simulink library "libturbines"  (R2025b)
settings: Solver=ode45  StartTime=0.0  StopTime=10.0  RelTol=1e-3  EnableMultiTasking=on
undefined symbols (not defined in the file): DiscIntNeverNeededParam, dt, faultOptions, noiseFlag
libraries: simulink x57, $bdroot x3
(part 1 of 5)
settings Model: Creator=grunnet  LastModifiedBy=yerai
settings SolverCC: AlgebraicLoopSolver=TrustRegion
settings DataIOCC: LimitDataPoints=on  SaveFormat=Array  SignalLoggingSaveFormat=ModelDataLogs  ReturnWorkspaceOutputs=off
settings OptimizationCC: ExpressionDepthLimit=2147483647.0  LifeSpan=inf
settings DebuggingCC: UnderspecifiedInitializationDetection=Classic  MergeDetectMultiDrivingBlocksExec=none  SolverPrmCheckMsg=warning  FcnCallInpInsideContextMsg=warning  UnconnectedInputMsg=warning  UnconnectedOutputMsg=warning  UnconnectedLineMsg=warning  StateNameClashWarn=warning  SFUnexpectedBacktrackingDiag=warning  SFNoUnconditionalDefaultTransitionDiag=warning  SFExecutionAtInitializationDiag=none  ArithmeticOperatorsInVariantConditions=warning
settings HardwareCC: ProdBitPerPointer=32.0  ProdBitPerSizeT=32.0  ProdBitPerPtrDiffT=32.0  ProdLargestAtomicFloat=None  ProdIntDivRoundTo=Undefined  ProdEndianess=Unspecified  ProdWordSize=32.0  ProdHWDeviceType=32-bit Generic
settings ModelReferenceCC: EnableRefExpFcnMdlSchedulingChecks=on  PropagateSignalLabelsOutOfModel=off
settings SFSimCC: SimUseLocalCustomCode=off  CustomCodeUndefinedFunction=UseInterfaceOnly
settings RTWCC: RTWUseLocalCustomCode=off  GPUComputeCapability=3.5  DLArmComputeVersion=19.05
settings CodeAppCC: StateflowObjectComments=on
settings GRTTargetCC: TargetLangStandard=C89/C90 (ANSI)  CombineOutputUpdateFcns=off  GRTInterface=on
settings ConfigComp: CovMetricSettings=dw  CovSaveCumulativeToWorkspaceVar=on  CovSaveSingleToWorkspaceVar=on  CovExternalEMLEnable=off

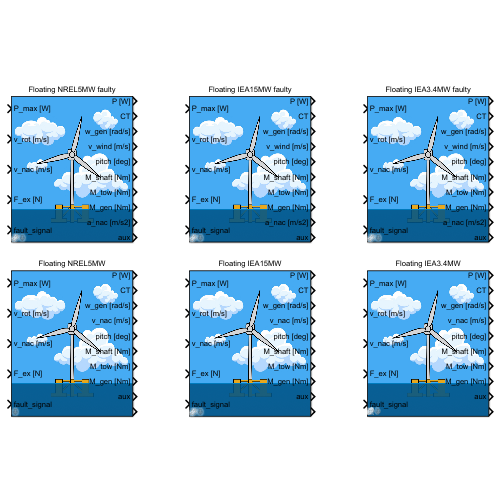
[thumbnail: Simulink's stored preview of the top-level diagram]
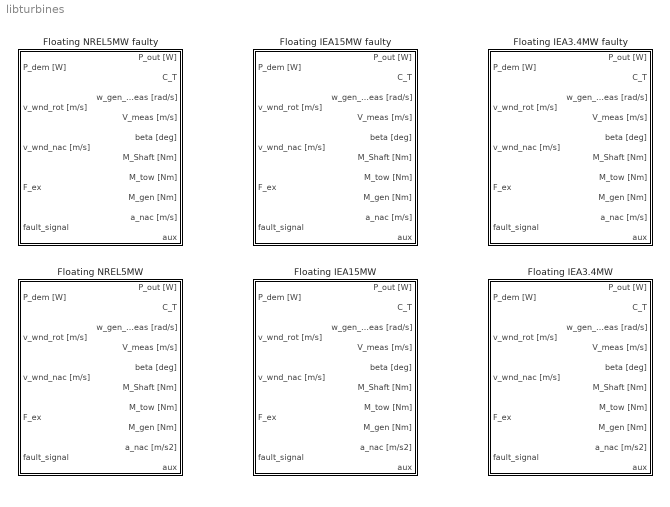
== system libturbines ==
  Floating IEA15MW : Subsystem  AncestorBlock=libturbines/Floating NREL5MW  mask(Wind Turbine){w_gen_ini=0.78788, beta_ini=0, auto=on, torq_ini=0}
      mask prompts: w_gen_ini "Initial generator velocity  [rad/s]"; beta_ini "Initial blade pitch [degrees]"; auto "Auto initial torque"; torq_ini "Initial generator torque"
      mask help: NREL 5MW Virtual Turbine
      mask init:
      | % l = load(file);
      | l               = get_param(gcb,'UserData');
      | env             = l.env;
      | wt              = l.wt;
      | plat            = l.plat;
      | wt.ctrl.gen.ini = w_gen_ini;
      | 
      | 
      | if(auto)
      |     wt.ctrl.torq.ini = min(interp1(wt.ctrl.torq.wg,wt.ctrl.torq.M,w_gen_ini,'spline'),wt.ctrl.torq.lim);
      | else
      |     wt.ctrl.torq.ini = torq_ini;
      | end
      | 
      | wt.pitch.ini        = beta_ini;
      | wt.ctrl.pitch.ini   = beta_ini;
      | wt.gen.torq.ini     = wt.ctrl.torq.ini;
      | wt.gen.ini          = w_gen_ini;
      | wt.rotor.ini        = w_gen_ini/wt.gen.N;
      mask Display:
      | image('FOWT.png');
      | 
      | port_label('output',1,'P [W]')
      | port_label('output',2,'CT')
      | port_label('output',3,'w_gen [rad/s]')
      | port_label('output',4,'v_nac [m/s]')
      | port_label('output',5,'pitch [deg]')
      | port_label('output',6,'M_shaft [Nm]')
      | port_label('output',7,'M_tow [Nm]')
      | port_label('output',8,'M_gen [Nm]')
      | port_label('output',9,'aux')
      | 
      | port_label('input',1,'P_max [W]')
      | port_label('input',2,'v_rot [m/s]')
      | port_label('input',3,'v_nac [m/s]')
      | port_label('input',4,'F_ex [N]')
      | port_label('input',5,'fault_signal')
  Floating IEA15MW faulty : Subsystem  AncestorBlock=libturbines/Floating NREL5MW faulty  mask(Wind Turbine){w_gen_ini=0.78788, beta_ini=0, auto=on, torq_ini=0}
      mask prompts: w_gen_ini "Initial generator velocity  [rad/s]"; beta_ini "Initial blade pitch [degrees]"; auto "Auto initial torque"; torq_ini "Initial generator torque"
      mask help: NREL 5MW Virtual Turbine
      mask init: same as libturbines/Floating IEA15MW
      mask Display:
      | image('FOWT.png');
      | 
      | port_label('output',1,'P [W]')
      | port_label('output',2,'CT')
      | port_label('output',3,'w_gen [rad/s]')
      | port_label('output',4,'v_wind [m/s]')
      | port_label('output',5,'pitch [deg]')
      | port_label('output',6,'M_shaft [Nm]')
      | port_label('output',7,'M_tow [Nm]')
      | port_label('output',8,'M_gen [Nm]')
      | port_label('output',9,'a_nac [m/s2]')
      | port_label('output',10,'aux')
      | 
      | port_label('input',1,'P_max [W]')
      | port_label('input',2,'v_rot [m/s]')
      | port_label('input',3,'v_nac [m/s]')
      | port_label('input',4,'F_ex [N]')
      | port_label('input',5,'fault_signal')
  Floating IEA3.4MW : Subsystem  AncestorBlock=libturbines/Floating IEA15MW  mask(Wind Turbine){w_gen_ini=118.1754, beta_ini=0, auto=on, torq_ini=0}
      mask prompts: w_gen_ini "Initial generator velocity  [rad/s]"; beta_ini "Initial blade pitch [degrees]"; auto "Auto initial torque"; torq_ini "Initial generator torque"
      mask help: NREL 5MW Virtual Turbine
      mask init: same as libturbines/Floating IEA15MW
      mask Display:
      | image('FOWT.png');
      | 
      | port_label('output',1,'P [W]')
      | port_label('output',2,'CT')
      | port_label('output',3,'w_gen [rad/s]')
      | port_label('output',4,'v_nac [m/s]')
      | port_label('output',5,'pitch [deg]')
      | port_label('output',6,'M_shaft [Nm]')
      | port_label('output',7,'M_tow [Nm]')
      | port_label('output',8,'M_gen [Nm]')
      | port_label('output',9,'aux')
      | 
      | port_label('input',1,'P_max [W]')
      | port_label('input',2,'v_rot [m/s]')
      | port_label('input',3,'v_nac [m/s]')
      | port_label('input',4,'F_ex [N]')
      | port_label('input',5,'fault_signal')
  Floating IEA3.4MW faulty : Subsystem  AncestorBlock=libturbines/Floating IEA15MW faulty  mask(Wind Turbine){w_gen_ini=118.1754, beta_ini=0, auto=on, torq_ini=0}
      mask prompts: w_gen_ini "Initial generator velocity  [rad/s]"; beta_ini "Initial blade pitch [degrees]"; auto "Auto initial torque"; torq_ini "Initial generator torque"
      mask help: NREL 5MW Virtual Turbine
      mask init: same as libturbines/Floating IEA15MW
      mask Display:
      | image('FOWT.png');
      | 
      | port_label('output',1,'P [W]')
      | port_label('output',2,'CT')
      | port_label('output',3,'w_gen [rad/s]')
      | port_label('output',4,'v_wind [m/s]')
      | port_label('output',5,'pitch [deg]')
      | port_label('output',6,'M_shaft [Nm]')
      | port_label('output',7,'M_tow [Nm]')
      | port_label('output',8,'M_gen [Nm]')
      | port_label('output',9,'a_nac [m/s2]')
      | port_label('output',10,'aux')
      | 
      | port_label('input',1,'P_max [W]')
      | port_label('input',2,'v_rot [m/s]')
      | port_label('input',3,'v_nac [m/s]')
      | port_label('input',4,'F_ex [N]')
      | port_label('input',5,'fault_signal')
  Floating NREL5MW : Subsystem  mask(Wind Turbine){w_gen_ini=50, beta_ini=0, auto=off, torq_ini=0}
      mask prompts: w_gen_ini "Initial generator velocity  [rad/s]"; beta_ini "Initial blade pitch [degrees]"; auto "Auto initial torque"; torq_ini "Initial generator torque"
      mask help: NREL 5MW Virtual Turbine
      mask init: same as libturbines/Floating IEA15MW
      mask Display:
      | image('FOWT.png');
      | 
      | port_label('output',1,'P [W]')
      | port_label('output',2,'CT')
      | port_label('output',3,'w_gen [rad/s]')
      | port_label('output',4,'v_nac [m/s]')
      | port_label('output',5,'pitch [deg]')
      | port_label('output',6,'M_shaft [Nm]')
      | port_label('output',7,'M_tow [Nm]')
      | port_label('output',8,'M_gen [Nm]')
      | port_label('output',9,'aux')
      | 
      | port_label('input',1,'P_max [W]')
      | port_label('input',2,'v_rot [m/s]')
      | port_label('input',3,'v_nac [m/s]')
      | port_label('input',4,'F_ex [N]')
      | port_label('input',5,'fault_signal')
  Floating NREL5MW faulty : Subsystem  AncestorBlock=libturbines/Faulty NREL5MW  mask(Wind Turbine){w_gen_ini=50, beta_ini=0, auto=off, torq_ini=0}
      mask prompts: w_gen_ini "Initial generator velocity  [rad/s]"; beta_ini "Initial blade pitch [degrees]"; auto "Auto initial torque"; torq_ini "Initial generator torque"
      mask help: NREL 5MW Virtual Turbine
      mask init: same as libturbines/Floating IEA15MW
      mask Display:
      | image('FOWT.png');
      | 
      | port_label('output',1,'P [W]')
      | port_label('output',2,'CT')
      | port_label('output',3,'w_gen [rad/s]')
      | port_label('output',4,'v_wind [m/s]')
      | port_label('output',5,'pitch [deg]')
      | port_label('output',6,'M_shaft [Nm]')
      | port_label('output',7,'M_tow [Nm]')
      | port_label('output',8,'M_gen [Nm]')
      | port_label('output',9,'a_nac [m/s2]')
      | port_label('output',10,'aux')
      | 
      | port_label('input',1,'P_max [W]')
      | port_label('input',2,'v_rot [m/s]')
      | port_label('input',3,'v_nac [m/s]')
      | port_label('input',4,'F_ex [N]')
      | port_label('input',5,'fault_signal')

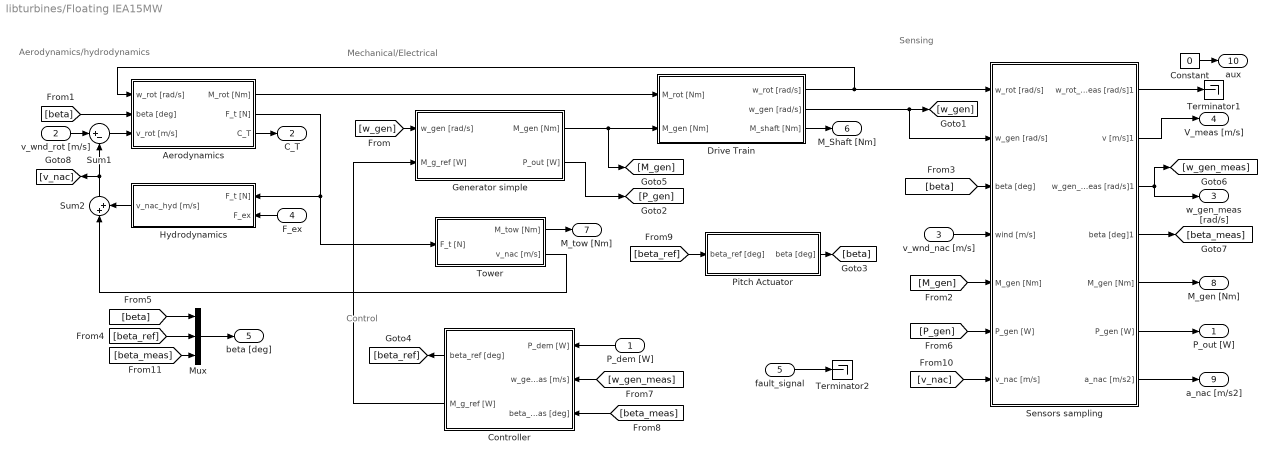
== system libturbines/Floating IEA15MW ==
  note: Control
  note: Aerodynamics/hydrodynamics
  note: Mechanical/Electrical
  note: Sensing
  P_dem [W] : Inport
  v_wnd_rot [m/s] : Inport  Port=2
  v_wnd_nac [m/s] : Inport  Port=3
  F_ex : Inport  Port=4
  fault_signal : Inport  Port=5
  Aerodynamics : Subsystem
  Constant : Constant  Value=0
  Controller : Subsystem
  Drive Train : Subsystem
  Generator simple : Subsystem
  Hydrodynamics : Subsystem
  Mux : Mux  Inputs=3
  Pitch Actuator : Subsystem
  Sensors sampling : Subsystem
  Sum1 : Sum  Inputs=|+-  InputSameDT=on  SaturateOnIntegerOverflow=on  OutDataTypeStr=Inherit: Same as first input
  Sum2 : Sum  Inputs=|++  InputSameDT=on  SaturateOnIntegerOverflow=on  OutDataTypeStr=Inherit: Same as first input
  Terminator1 : Terminator
  Terminator2 : Terminator
  "Tower " : Subsystem
  P_out [W] : Outport
  C_T : Outport  Port=2
  w_gen_meas [rad/s] : Outport  Port=3
  V_meas [m/s] : Outport  Port=4
  beta [deg] : Outport  Port=5
  M_Shaft [Nm] : Outport  Port=6
  M_tow [Nm] : Outport  Port=7
  M_gen [Nm] : Outport  Port=8
  a_nac [m/s2] : Outport  Port=9
  aux : Outport  Port=10
  wires:
  Sensors sampling/7(a_nac [m/s2]) -> a_nac [m/s2]/1
  [v_nac] -> Sensors sampling/7("v_nac [m/s] ")
  "Tower "/2(v_nac [m/s]) -> Sum2/1
  Sum2/1 -> Sum1/2, [v_nac]
  Hydrodynamics/1(v_nac_hyd [m/s]) -> Sum2/2
  [P_gen] -> Sensors sampling/6("P_gen [W] ")
  [M_gen] -> Sensors sampling/5("M_gen [Nm] ")
  Generator simple/2(P_out [W]) -> [P_gen]
  Sensors sampling/6(P_gen [W]) -> P_out [W]/1
  Sensors sampling/5(M_gen [Nm]) -> M_gen [Nm]/1
  Sensors sampling/4(beta [deg]1) -> [beta_meas]
  Sensors sampling/3(w_gen_meas [rad/s]1) -> [w_gen_meas], w_gen_meas [rad/s]/1
  Sensors sampling/2(v [m/s]1) -> V_meas [m/s]/1
  Sensors sampling/1(w_rot_meas [rad/s]1) -> Terminator1/1
  [beta] -> Aerodynamics/2(beta [deg])
  [w_gen] -> Generator simple/1(w_gen [rad/s])
  fault_signal/1 -> Terminator2/1
  Drive Train/3(M_shaft [Nm]) -> M_Shaft [Nm]/1
  v_wnd_nac [m/s]/1 -> Sensors sampling/4(wind [m/s])
  v_wnd_rot [m/s]/1 -> Sum1/1
  "Tower "/1(M_tow [Nm]) -> M_tow [Nm]/1
  Aerodynamics/2(F_t [N]) -> Hydrodynamics/1(F_t [N]), "Tower "/1(F_t [N])
  Pitch Actuator/1(beta [deg]) -> [beta]
  Controller/1(beta_ref [deg]) -> [beta_ref]
  P_dem [W]/1 -> Controller/1(P_dem [W])
  Controller/2(M_g_ref [W]) -> Generator simple/2(M_g_ref [W])
  Sum1/1 -> Aerodynamics/3(v_rot [m/s])
  Drive Train/2(w_gen [rad/s]) -> [w_gen], Sensors sampling/2(w_gen [rad/s])
  Generator simple/1(M_gen [Nm]) -> Drive Train/2(M_gen [Nm]), [M_gen]
  Drive Train/1(w_rot [rad/s]) -> Aerodynamics/1(w_rot [rad/s]), Sensors sampling/1("w_rot [rad/s] ")
  Aerodynamics/1(M_rot [Nm]) -> Drive Train/1(M_rot [Nm])
  Aerodynamics/3(C_T) -> C_T/1
  [beta] -> Sensors sampling/3("beta [deg] ")
  [beta_ref] -> Mux/2
  [beta] -> Mux/1
  [w_gen_meas] -> Controller/2(w_gen_meas [m/s])
  [beta_meas] -> Controller/3(beta_meas [deg])
  [beta_ref] -> Pitch Actuator/1(beta_ref [deg])
  [beta_meas] -> Mux/3
  F_ex/1 -> Hydrodynamics/2(F_ex)
  Mux/1 -> beta [deg]/1
  Constant/1 -> aux/1

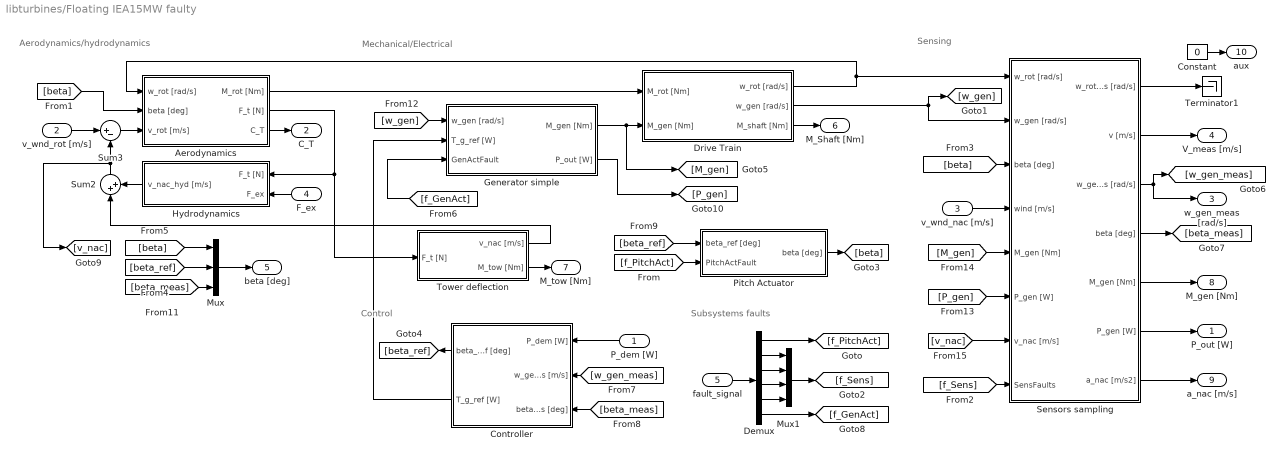
== system libturbines/Floating IEA15MW faulty ==
  note: Subsystems faults
  note: Sensing
  note: Mechanical/Electrical
  note: Aerodynamics/hydrodynamics
  note: Control
  P_dem [W] : Inport
  v_wnd_rot [m/s] : Inport  Port=2
  v_wnd_nac [m/s] : Inport  Port=3
  F_ex : Inport  Port=4
  fault_signal : Inport  Port=5
  Aerodynamics : Subsystem
  Constant : Constant  Value=0
  Controller : Subsystem
  Demux : Demux  Outputs=6
  Drive Train : Subsystem
  Generator simple : Subsystem
  Hydrodynamics : Subsystem
  Mux : Mux  Inputs=3
  Mux1 : Mux
  Pitch Actuator : Subsystem
  Sensors sampling : Subsystem
  Sum2 : Sum  Inputs=|++  InputSameDT=on  SaturateOnIntegerOverflow=on  OutDataTypeStr=Inherit: Same as first input
  Sum3 : Sum  Inputs=|+-  InputSameDT=on  SaturateOnIntegerOverflow=on  OutDataTypeStr=Inherit: Same as first input
  Terminator1 : Terminator
  "Tower deflection " : Subsystem
  P_out [W] : Outport
  C_T : Outport  Port=2
  w_gen_meas [rad/s] : Outport  Port=3
  V_meas [m/s] : Outport  Port=4
  beta [deg] : Outport  Port=5
  M_Shaft [Nm] : Outport  Port=6
  M_tow [Nm] : Outport  Port=7
  M_gen [Nm] : Outport  Port=8
  a_nac [m/s] : Outport  Port=9
  aux : Outport  Port=10
  wires:
  Demux/5 -> Mux1/4
  Demux/6 -> [f_GenAct]
  Sensors sampling/7(a_nac [m/s2]) -> a_nac [m/s]/1
  [v_nac] -> Sensors sampling/7("v_nac [m/s] ")
  "Tower deflection "/1(v_nac [m/s]) -> Sum2/1
  Sum2/1 -> Sum3/2, [v_nac]
  Hydrodynamics/1(v_nac_hyd [m/s]) -> Sum2/2
  v_wnd_rot [m/s]/1 -> Sum3/1
  Sum3/1 -> Aerodynamics/3(v_rot [m/s])
  [M_gen] -> Sensors sampling/5("M_gen [Nm] ")
  [P_gen] -> Sensors sampling/6("P_gen [W] ")
  Generator simple/2(P_out [W]) -> [P_gen]
  Sensors sampling/5(M_gen [Nm]) -> M_gen [Nm]/1
  Sensors sampling/6(P_gen [W]) -> P_out [W]/1
  [w_gen] -> Generator simple/1(w_gen [rad/s])
  [beta] -> Aerodynamics/2(beta [deg])
  Mux1/1 -> [f_Sens]
  Demux/4 -> Mux1/3
  Demux/2 -> Mux1/1
  Demux/3 -> Mux1/2
  Constant/1 -> aux/1
  Mux/1 -> beta [deg]/1
  F_ex/1 -> Hydrodynamics/2(F_ex)
  [beta_meas] -> Mux/3
  [beta_ref] -> Pitch Actuator/1(beta_ref [deg])
  [beta_meas] -> Controller/3(beta_meas [deg])
  [w_gen_meas] -> Controller/2(w_gen_meas [m/s])
  [f_GenAct] -> Generator simple/3(GenActFault)
  [beta] -> Mux/1
  [beta_ref] -> Mux/2
  [beta] -> Sensors sampling/3("beta [deg] ")
  [f_Sens] -> Sensors sampling/8(SensFaults)
  [f_PitchAct] -> Pitch Actuator/2(PitchActFault)
  Demux/1 -> [f_PitchAct]
  fault_signal/1 -> Demux/1
  Aerodynamics/3(C_T) -> C_T/1
  Aerodynamics/1(M_rot [Nm]) -> Drive Train/1(M_rot [Nm])
  Drive Train/1(w_rot [rad/s]) -> Sensors sampling/1("w_rot [rad/s] "), Aerodynamics/1(w_rot [rad/s])
  Generator simple/1(M_gen [Nm]) -> Drive Train/2(M_gen [Nm]), [M_gen]
  Drive Train/2(w_gen [rad/s]) -> Sensors sampling/2(w_gen [rad/s]), [w_gen]
  Sensors sampling/4(beta [deg]) -> [beta_meas]
  Sensors sampling/2(v [m/s]) -> V_meas [m/s]/1
  Controller/2(T_g_ref [W]) -> Generator simple/2(T_g_ref [W])
  Sensors sampling/3(w_gen_meas [rad/s]) -> [w_gen_meas], w_gen_meas [rad/s]/1
  P_dem [W]/1 -> Controller/1(P_dem [W])
  Controller/1(beta_ref [deg]) -> [beta_ref]
  Pitch Actuator/1(beta [deg]) -> [beta]
  Aerodynamics/2(F_t [N]) -> Hydrodynamics/1(F_t [N]), "Tower deflection "/1(F_t [N])
  "Tower deflection "/2(M_tow [Nm]) -> M_tow [Nm]/1
  v_wnd_nac [m/s]/1 -> Sensors sampling/4(wind [m/s])
  Drive Train/3(M_shaft [Nm]) -> M_Shaft [Nm]/1
  Sensors sampling/1(w_rot_meas [rad/s]) -> Terminator1/1

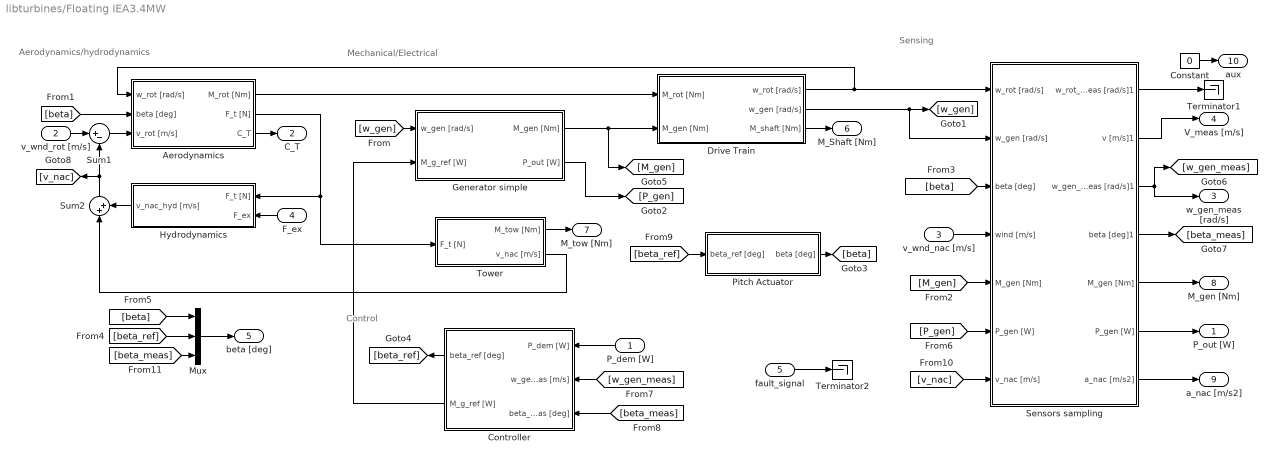
== system libturbines/Floating IEA3.4MW ==
  note: Control
  note: Aerodynamics/hydrodynamics
  note: Mechanical/Electrical
  note: Sensing
  P_dem [W] : Inport
  v_wnd_rot [m/s] : Inport  Port=2
  v_wnd_nac [m/s] : Inport  Port=3
  F_ex : Inport  Port=4
  fault_signal : Inport  Port=5
  Aerodynamics : Subsystem
  Constant : Constant  Value=0
  Controller : Subsystem
  Drive Train : Subsystem
  Generator simple : Subsystem
  Hydrodynamics : Subsystem
  Mux : Mux  Inputs=3
  Pitch Actuator : Subsystem
  Sensors sampling : Subsystem
  Sum1 : Sum  Inputs=|+-  InputSameDT=on  SaturateOnIntegerOverflow=on  OutDataTypeStr=Inherit: Same as first input
  Sum2 : Sum  Inputs=|++  InputSameDT=on  SaturateOnIntegerOverflow=on  OutDataTypeStr=Inherit: Same as first input
  Terminator1 : Terminator
  Terminator2 : Terminator
  "Tower " : Subsystem
  P_out [W] : Outport
  C_T : Outport  Port=2
  w_gen_meas [rad/s] : Outport  Port=3
  V_meas [m/s] : Outport  Port=4
  beta [deg] : Outport  Port=5
  M_Shaft [Nm] : Outport  Port=6
  M_tow [Nm] : Outport  Port=7
  M_gen [Nm] : Outport  Port=8
  a_nac [m/s2] : Outport  Port=9
  aux : Outport  Port=10
  wires:
  Sensors sampling/7(a_nac [m/s2]) -> a_nac [m/s2]/1
  [v_nac] -> Sensors sampling/7("v_nac [m/s] ")
  "Tower "/2(v_nac [m/s]) -> Sum2/1
  Sum2/1 -> Sum1/2, [v_nac]
  Hydrodynamics/1(v_nac_hyd [m/s]) -> Sum2/2
  [P_gen] -> Sensors sampling/6("P_gen [W] ")
  [M_gen] -> Sensors sampling/5("M_gen [Nm] ")
  Generator simple/2(P_out [W]) -> [P_gen]
  Sensors sampling/6(P_gen [W]) -> P_out [W]/1
  Sensors sampling/5(M_gen [Nm]) -> M_gen [Nm]/1
  Sensors sampling/4(beta [deg]1) -> [beta_meas]
  Sensors sampling/3(w_gen_meas [rad/s]1) -> [w_gen_meas], w_gen_meas [rad/s]/1
  Sensors sampling/2(v [m/s]1) -> V_meas [m/s]/1
  Sensors sampling/1(w_rot_meas [rad/s]1) -> Terminator1/1
  [beta] -> Aerodynamics/2(beta [deg])
  [w_gen] -> Generator simple/1(w_gen [rad/s])
  fault_signal/1 -> Terminator2/1
  Drive Train/3(M_shaft [Nm]) -> M_Shaft [Nm]/1
  v_wnd_nac [m/s]/1 -> Sensors sampling/4(wind [m/s])
  v_wnd_rot [m/s]/1 -> Sum1/1
  "Tower "/1(M_tow [Nm]) -> M_tow [Nm]/1
  Aerodynamics/2(F_t [N]) -> Hydrodynamics/1(F_t [N]), "Tower "/1(F_t [N])
  Pitch Actuator/1(beta [deg]) -> [beta]
  Controller/1(beta_ref [deg]) -> [beta_ref]
  P_dem [W]/1 -> Controller/1(P_dem [W])
  Controller/2(M_g_ref [W]) -> Generator simple/2(M_g_ref [W])
  Sum1/1 -> Aerodynamics/3(v_rot [m/s])
  Drive Train/2(w_gen [rad/s]) -> [w_gen], Sensors sampling/2(w_gen [rad/s])
  Generator simple/1(M_gen [Nm]) -> Drive Train/2(M_gen [Nm]), [M_gen]
  Drive Train/1(w_rot [rad/s]) -> Aerodynamics/1(w_rot [rad/s]), Sensors sampling/1("w_rot [rad/s] ")
  Aerodynamics/1(M_rot [Nm]) -> Drive Train/1(M_rot [Nm])
  Aerodynamics/3(C_T) -> C_T/1
  [beta] -> Sensors sampling/3("beta [deg] ")
  [beta_ref] -> Mux/2
  [beta] -> Mux/1
  [w_gen_meas] -> Controller/2(w_gen_meas [m/s])
  [beta_meas] -> Controller/3(beta_meas [deg])
  [beta_ref] -> Pitch Actuator/1(beta_ref [deg])
  [beta_meas] -> Mux/3
  F_ex/1 -> Hydrodynamics/2(F_ex)
  Mux/1 -> beta [deg]/1
  Constant/1 -> aux/1

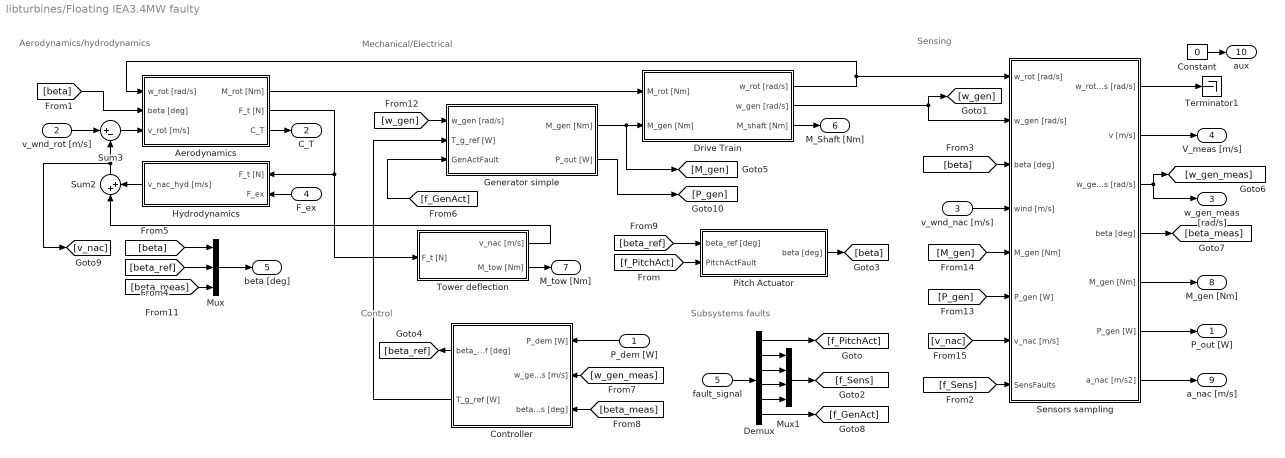
== system libturbines/Floating IEA3.4MW faulty ==
  note: Subsystems faults
  note: Sensing
  note: Mechanical/Electrical
  note: Aerodynamics/hydrodynamics
  note: Control
  P_dem [W] : Inport
  v_wnd_rot [m/s] : Inport  Port=2
  v_wnd_nac [m/s] : Inport  Port=3
  F_ex : Inport  Port=4
  fault_signal : Inport  Port=5
  Aerodynamics : Subsystem
  Constant : Constant  Value=0
  Controller : Subsystem
  Demux : Demux  Outputs=6
  Drive Train : Subsystem
  Generator simple : Subsystem
  Hydrodynamics : Subsystem
  Mux : Mux  Inputs=3
  Mux1 : Mux
  Pitch Actuator : Subsystem
  Sensors sampling : Subsystem
  Sum2 : Sum  Inputs=|++  InputSameDT=on  SaturateOnIntegerOverflow=on  OutDataTypeStr=Inherit: Same as first input
  Sum3 : Sum  Inputs=|+-  InputSameDT=on  SaturateOnIntegerOverflow=on  OutDataTypeStr=Inherit: Same as first input
  Terminator1 : Terminator
  "Tower deflection " : Subsystem
  P_out [W] : Outport
  C_T : Outport  Port=2
  w_gen_meas [rad/s] : Outport  Port=3
  V_meas [m/s] : Outport  Port=4
  beta [deg] : Outport  Port=5
  M_Shaft [Nm] : Outport  Port=6
  M_tow [Nm] : Outport  Port=7
  M_gen [Nm] : Outport  Port=8
  a_nac [m/s] : Outport  Port=9
  aux : Outport  Port=10
  wires:
  Demux/5 -> Mux1/4
  Demux/6 -> [f_GenAct]
  Sensors sampling/7(a_nac [m/s2]) -> a_nac [m/s]/1
  [v_nac] -> Sensors sampling/7("v_nac [m/s] ")
  "Tower deflection "/1(v_nac [m/s]) -> Sum2/1
  Sum2/1 -> Sum3/2, [v_nac]
  Hydrodynamics/1(v_nac_hyd [m/s]) -> Sum2/2
  v_wnd_rot [m/s]/1 -> Sum3/1
  Sum3/1 -> Aerodynamics/3(v_rot [m/s])
  [M_gen] -> Sensors sampling/5("M_gen [Nm] ")
  [P_gen] -> Sensors sampling/6("P_gen [W] ")
  Generator simple/2(P_out [W]) -> [P_gen]
  Sensors sampling/5(M_gen [Nm]) -> M_gen [Nm]/1
  Sensors sampling/6(P_gen [W]) -> P_out [W]/1
  [w_gen] -> Generator simple/1(w_gen [rad/s])
  [beta] -> Aerodynamics/2(beta [deg])
  Mux1/1 -> [f_Sens]
  Demux/4 -> Mux1/3
  Demux/2 -> Mux1/1
  Demux/3 -> Mux1/2
  Constant/1 -> aux/1
  Mux/1 -> beta [deg]/1
  F_ex/1 -> Hydrodynamics/2(F_ex)
  [beta_meas] -> Mux/3
  [beta_ref] -> Pitch Actuator/1(beta_ref [deg])
  [beta_meas] -> Controller/3(beta_meas [deg])
  [w_gen_meas] -> Controller/2(w_gen_meas [m/s])
  [f_GenAct] -> Generator simple/3(GenActFault)
  [beta] -> Mux/1
  [beta_ref] -> Mux/2
  [beta] -> Sensors sampling/3("beta [deg] ")
  [f_Sens] -> Sensors sampling/8(SensFaults)
  [f_PitchAct] -> Pitch Actuator/2(PitchActFault)
  Demux/1 -> [f_PitchAct]
  fault_signal/1 -> Demux/1
  Aerodynamics/3(C_T) -> C_T/1
  Aerodynamics/1(M_rot [Nm]) -> Drive Train/1(M_rot [Nm])
  Drive Train/1(w_rot [rad/s]) -> Sensors sampling/1("w_rot [rad/s] "), Aerodynamics/1(w_rot [rad/s])
  Generator simple/1(M_gen [Nm]) -> Drive Train/2(M_gen [Nm]), [M_gen]
  Drive Train/2(w_gen [rad/s]) -> Sensors sampling/2(w_gen [rad/s]), [w_gen]
  Sensors sampling/4(beta [deg]) -> [beta_meas]
  Sensors sampling/2(v [m/s]) -> V_meas [m/s]/1
  Controller/2(T_g_ref [W]) -> Generator simple/2(T_g_ref [W])
  Sensors sampling/3(w_gen_meas [rad/s]) -> [w_gen_meas], w_gen_meas [rad/s]/1
  P_dem [W]/1 -> Controller/1(P_dem [W])
  Controller/1(beta_ref [deg]) -> [beta_ref]
  Pitch Actuator/1(beta [deg]) -> [beta]
  Aerodynamics/2(F_t [N]) -> Hydrodynamics/1(F_t [N]), "Tower deflection "/1(F_t [N])
  "Tower deflection "/2(M_tow [Nm]) -> M_tow [Nm]/1
  v_wnd_nac [m/s]/1 -> Sensors sampling/4(wind [m/s])
  Drive Train/3(M_shaft [Nm]) -> M_Shaft [Nm]/1
  Sensors sampling/1(w_rot_meas [rad/s]) -> Terminator1/1

== system libturbines/Floating NREL5MW ==
  note: Sensing
  note: Mechanical/Electrical
  note: Aerodynamics/hydrodynamics
  note: Control
  P_dem [W] : Inport
  v_wnd_rot [m/s] : Inport  Port=2
  v_wnd_nac [m/s] : Inport  Port=3
  F_ex : Inport  Port=4
  fault_signal : Inport  Port=5
  Aerodynamics : Subsystem
  Constant : Constant  Value=0
  Controller : Subsystem
  Drive Train : Subsystem
  Generator simple : Subsystem
  Hydrodynamics : Subsystem
  Mux : Mux  Inputs=3
  Pitch Actuator : Subsystem
  Sensors sampling : Subsystem
  Sum1 : Sum  Inputs=|+-  InputSameDT=on  SaturateOnIntegerOverflow=on  OutDataTypeStr=Inherit: Same as first input
  Sum2 : Sum  Inputs=|++  InputSameDT=on  SaturateOnIntegerOverflow=on  OutDataTypeStr=Inherit: Same as first input
  Terminator1 : Terminator
  Terminator2 : Terminator
  "Tower " : Subsystem
  P_out [W] : Outport
  C_T : Outport  Port=2
  w_gen_meas [rad/s] : Outport  Port=3
  V_meas [m/s] : Outport  Port=4
  beta [deg] : Outport  Port=5
  M_Shaft [Nm] : Outport  Port=6
  M_tow [Nm] : Outport  Port=7
  M_gen [Nm] : Outport  Port=8
  a_nac [m/s2] : Outport  Port=9
  aux : Outport  Port=10
  wires:
  Constant/1 -> aux/1
  Mux/1 -> beta [deg]/1
  F_ex/1 -> Hydrodynamics/2(F_ex)
  [beta_meas] -> Mux/3
  [beta_ref] -> Pitch Actuator/1(beta_ref [deg])
  [beta_meas] -> Controller/3(beta_meas [deg])
  [w_gen_meas] -> Controller/2(w_gen_meas [m/s])
  [beta] -> Mux/1
  [beta_ref] -> Mux/2
  [beta] -> Sensors sampling/3("beta [deg] ")
  Aerodynamics/3(C_T) -> C_T/1
  Aerodynamics/1(M_rot [Nm]) -> Drive Train/1(M_rot [Nm])
  Drive Train/1(w_rot [rad/s]) -> Sensors sampling/1("w_rot [rad/s] "), Aerodynamics/1(w_rot [rad/s])
  Generator simple/1(M_gen [Nm]) -> [M_gen], Drive Train/2(M_gen [Nm])
  Drive Train/2(w_gen [rad/s]) -> Sensors sampling/2(w_gen [rad/s]), [w_gen]
  Sum1/1 -> Aerodynamics/3(v_rot [m/s])
  Controller/2(M_g_ref [W]) -> Generator simple/2(M_g_ref [W])
  P_dem [W]/1 -> Controller/1(P_dem [W])
  Controller/1(beta_ref [deg]) -> [beta_ref]
  Pitch Actuator/1(beta [deg]) -> [beta]
  Aerodynamics/2(F_t [N]) -> "Tower "/1(F_t [N]), Hydrodynamics/1(F_t [N])
  "Tower "/1(M_tow [Nm]) -> M_tow [Nm]/1
  v_wnd_rot [m/s]/1 -> Sum1/1
  v_wnd_nac [m/s]/1 -> Sensors sampling/4(wind [m/s])
  Drive Train/3(M_shaft [Nm]) -> M_Shaft [Nm]/1
  fault_signal/1 -> Terminator2/1
  [w_gen] -> Generator simple/1(w_gen [rad/s])
  [beta] -> Aerodynamics/2(beta [deg])
  Sensors sampling/1(w_rot_meas [rad/s]1) -> Terminator1/1
  Sensors sampling/2(v [m/s]1) -> V_meas [m/s]/1
  Sensors sampling/3(w_gen_meas [rad/s]1) -> w_gen_meas [rad/s]/1, [w_gen_meas]
  Sensors sampling/4(beta [deg]1) -> [beta_meas]
  Sensors sampling/5(M_gen [Nm]) -> M_gen [Nm]/1
  Sensors sampling/6(P_gen [W]) -> P_out [W]/1
  Generator simple/2(P_out [W]) -> [P_gen]
  [M_gen] -> Sensors sampling/5("M_gen [Nm] ")
  [P_gen] -> Sensors sampling/6("P_gen [W] ")
  Hydrodynamics/1(v_nac_hyd [m/s]) -> Sum2/2
  Sum2/1 -> [v_nac], Sum1/2
  "Tower "/2(v_nac [m/s]) -> Sum2/1
  [v_nac] -> Sensors sampling/7("v_nac [m/s] ")
  Sensors sampling/7(a_nac [m/s2]) -> a_nac [m/s2]/1

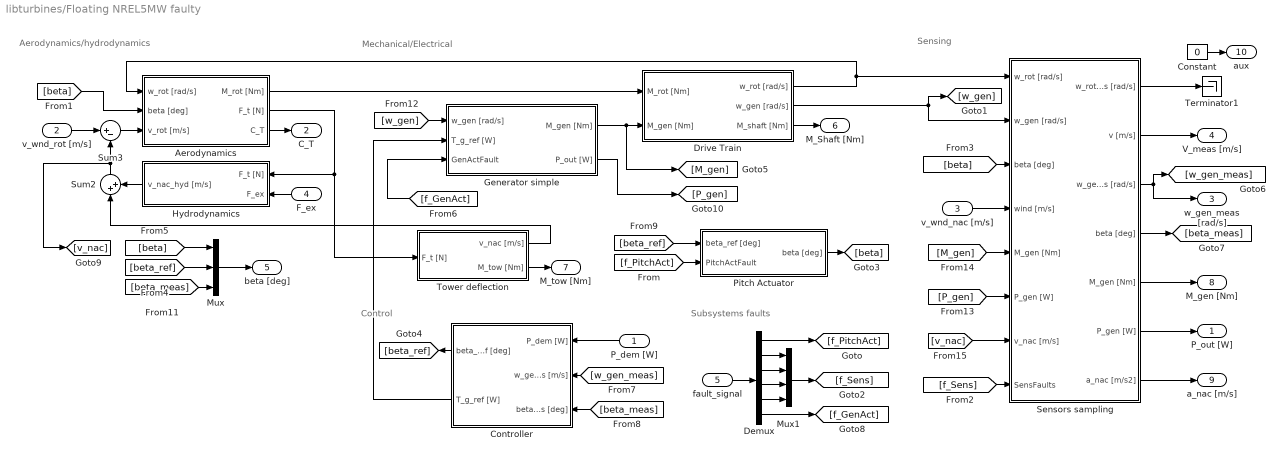
== system libturbines/Floating NREL5MW faulty ==
  note: Control
  note: Aerodynamics/hydrodynamics
  note: Mechanical/Electrical
  note: Sensing
  note: Subsystems faults
  P_dem [W] : Inport
  v_wnd_rot [m/s] : Inport  Port=2
  v_wnd_nac [m/s] : Inport  Port=3
  F_ex : Inport  Port=4
  fault_signal : Inport  Port=5
  Aerodynamics : Subsystem
  Constant : Constant  Value=0
  Controller : Subsystem
  Demux : Demux  Outputs=6
  Drive Train : Subsystem
  Generator simple : Subsystem
  Hydrodynamics : Subsystem
  Mux : Mux  Inputs=3
  Mux1 : Mux
  Pitch Actuator : Subsystem
  Sensors sampling : Subsystem
  Sum2 : Sum  Inputs=|++  InputSameDT=on  SaturateOnIntegerOverflow=on  OutDataTypeStr=Inherit: Same as first input
  Sum3 : Sum  Inputs=|+-  InputSameDT=on  SaturateOnIntegerOverflow=on  OutDataTypeStr=Inherit: Same as first input
  Terminator1 : Terminator
  "Tower deflection " : Subsystem
  P_out [W] : Outport
  C_T : Outport  Port=2
  w_gen_meas [rad/s] : Outport  Port=3
  V_meas [m/s] : Outport  Port=4
  beta [deg] : Outport  Port=5
  M_Shaft [Nm] : Outport  Port=6
  M_tow [Nm] : Outport  Port=7
  M_gen [Nm] : Outport  Port=8
  a_nac [m/s] : Outport  Port=9
  aux : Outport  Port=10
  wires:
  Sensors sampling/1(w_rot_meas [rad/s]) -> Terminator1/1
  Drive Train/3(M_shaft [Nm]) -> M_Shaft [Nm]/1
  v_wnd_nac [m/s]/1 -> Sensors sampling/4(wind [m/s])
  "Tower deflection "/2(M_tow [Nm]) -> M_tow [Nm]/1
  Aerodynamics/2(F_t [N]) -> "Tower deflection "/1(F_t [N]), Hydrodynamics/1(F_t [N])
  Pitch Actuator/1(beta [deg]) -> [beta]
  Controller/1(beta_ref [deg]) -> [beta_ref]
  P_dem [W]/1 -> Controller/1(P_dem [W])
  Sensors sampling/3(w_gen_meas [rad/s]) -> w_gen_meas [rad/s]/1, [w_gen_meas]
  Controller/2(T_g_ref [W]) -> Generator simple/2(T_g_ref [W])
  Sensors sampling/2(v [m/s]) -> V_meas [m/s]/1
  Sensors sampling/4(beta [deg]) -> [beta_meas]
  Drive Train/2(w_gen [rad/s]) -> [w_gen], Sensors sampling/2(w_gen [rad/s])
  Generator simple/1(M_gen [Nm]) -> [M_gen], Drive Train/2(M_gen [Nm])
  Drive Train/1(w_rot [rad/s]) -> Aerodynamics/1(w_rot [rad/s]), Sensors sampling/1("w_rot [rad/s] ")
  Aerodynamics/1(M_rot [Nm]) -> Drive Train/1(M_rot [Nm])
  Aerodynamics/3(C_T) -> C_T/1
  fault_signal/1 -> Demux/1
  Demux/1 -> [f_PitchAct]
  [f_PitchAct] -> Pitch Actuator/2(PitchActFault)
  [f_Sens] -> Sensors sampling/8(SensFaults)
  [beta] -> Sensors sampling/3("beta [deg] ")
  [beta_ref] -> Mux/2
  [beta] -> Mux/1
  [f_GenAct] -> Generator simple/3(GenActFault)
  [w_gen_meas] -> Controller/2(w_gen_meas [m/s])
  [beta_meas] -> Controller/3(beta_meas [deg])
  [beta_ref] -> Pitch Actuator/1(beta_ref [deg])
  [beta_meas] -> Mux/3
  F_ex/1 -> Hydrodynamics/2(F_ex)
  Mux/1 -> beta [deg]/1
  Constant/1 -> aux/1
  Demux/3 -> Mux1/2
  Demux/2 -> Mux1/1
  Demux/4 -> Mux1/3
  Mux1/1 -> [f_Sens]
  [beta] -> Aerodynamics/2(beta [deg])
  [w_gen] -> Generator simple/1(w_gen [rad/s])
  Sensors sampling/6(P_gen [W]) -> P_out [W]/1
  Sensors sampling/5(M_gen [Nm]) -> M_gen [Nm]/1
  Generator simple/2(P_out [W]) -> [P_gen]
  [P_gen] -> Sensors sampling/6("P_gen [W] ")
  [M_gen] -> Sensors sampling/5("M_gen [Nm] ")
  Sum3/1 -> Aerodynamics/3(v_rot [m/s])
  v_wnd_rot [m/s]/1 -> Sum3/1
  Hydrodynamics/1(v_nac_hyd [m/s]) -> Sum2/2
  Sum2/1 -> [v_nac], Sum3/2
  "Tower deflection "/1(v_nac [m/s]) -> Sum2/1
  [v_nac] -> Sensors sampling/7("v_nac [m/s] ")
  Sensors sampling/7(a_nac [m/s2]) -> a_nac [m/s]/1
  Demux/6 -> [f_GenAct]
  Demux/5 -> Mux1/4

== system libturbines/Floating IEA15MW/Aerodynamics ==
  note: tip speed
      | [m/s]
  w_rot [rad/s] : Inport
  beta [deg] : Inport  Port=2
  v_rot [m/s] : Inport  Port=3
  C_P & C_T tables1 : $bdroot/Floating NREL5MW faulty/Aerodynamics/Blade 1/C_P & C_T tables  SystemSampleTime=-1  VariantActivationTime=update diagram  EmptyChoice=off  PassThrough=off  PassThroughVariantControl=(default)  EmptyChoiceVariantControl=(default)  AllowFlexibleInterface=on  Latency=0  AutoFrameSizeCalculation=off
  Math Function : Math  Operator=square  SignedPower=on
  Product : Product  InputSameDT=on  SaturateOnIntegerOverflow=on  OutDataTypeStr=Inherit: Same as first input
  Product1 : Product  Inputs=**/  InputSameDT=on  SaturateOnIntegerOverflow=on  OutDataTypeStr=Inherit: Same as first input
  Product2 : Product  InputSameDT=on  SaturateOnIntegerOverflow=on  OutDataTypeStr=Inherit: Same as first input
  Product3 : Product  Inputs=/*  InputSameDT=on  SaturateOnIntegerOverflow=on  OutDataTypeStr=Inherit: Same as first input
  rho/2*A : Gain  Gain=env.rho*.5* pi * wt.rotor.radius^2  SaturateOnIntegerOverflow=on  OutDataTypeStr=Inherit: Same as input  ParamDataTypeStr=Inherit: Same as input
  rotor radius : Gain  Gain=wt.rotor.radius  SaturateOnIntegerOverflow=on  OutDataTypeStr=Inherit: Same as input  ParamDataTypeStr=Inherit: Same as input
  M_rot [Nm] : Outport
  F_t [N] : Outport  Port=2
  C_T : Outport  Port=3
  wires:
  rho/2*A/1 -> Product/1, Product2/2
  C_P & C_T tables1/1 -> Product/2, C_T/1
  Product3/1 -> C_P & C_T tables1/2
  w_rot [rad/s]/1 -> Product1/3, rotor radius/1
  v_rot [m/s]/1 -> Product2/1, Product3/1, Math Function/1
  Math Function/1 -> rho/2*A/1
  rotor radius/1 -> Product3/2
  C_P & C_T tables1/2 -> Product1/1
  beta [deg]/1 -> C_P & C_T tables1/1
  Product/1 -> F_t [N]/1
  Product1/1 -> M_rot [Nm]/1
  Product2/1 -> Product1/2

== system libturbines/Floating IEA15MW/Controller ==
  P_dem [W] : Inport
  w_gen_meas [m/s] : Inport  Port=2
  beta_meas [deg] : Inport  Port=3
  Generator efficiency compensation : Gain  Gain=1/wt.ctrl.gen.effeciency
  Limit power to rated : Saturate  UpperLimit=wt.ctrl.p_rated  LowerLimit=0
  Measurement filter (low pass) : DiscreteStateSpace  A=wt.ctrl.alpha  B=1-wt.ctrl.alpha  C=wt.ctrl.alpha  D=1-wt.ctrl.alpha  InitialCondition=wt.ctrl.gen.ini  SampleTime=wt.ctrl.Ts
  Pitch controller : Subsystem  TreatAsAtomicUnit=on
  Rate Limiter : RateLimiter  RisingSlewLimit=wt.ctrl.torq.ratelim  FallingSlewLimit=-wt.ctrl.torq.ratelim  SampleTimeMode=inherited  InitialCondition=wt.ctrl.torq.ini
  Rated speed : Constant  Value=wt.ctrl.gen.rated
  Region check : Subsystem
  Sample output : ZeroOrderHold  SampleTime=wt.ctrl.Ts
  Sample power demand : ZeroOrderHold  SampleTime=wt.ctrl.Ts
  Saturation : Saturate  UpperLimit=wt.ctrl.torq.lim  LowerLimit=0
  Sum : Sum  Inputs=+-|
  Torque - speed lookup table : Lookup  InputValues=wt.ctrl.torq.wg  Table=wt.ctrl.torq.M  LookUpMeth=Interpolation-Use End Values  SaturateOnIntegerOverflow=off
  Zero-Order Hold : ZeroOrderHold  SampleTime=wt.ctrl.Ts
  beta_ref [deg] : Outport
  M_g_ref [W] : Outport  Port=2
  wires:
  Region check/2(Enable pitch controller) -> Pitch controller/Enable
  Sum/1 -> Pitch controller/1(w_gen_diff)
  Rated speed/1 -> Sum/1
  Sample power demand/1 -> Generator efficiency compensation/1
  Rate Limiter/1 -> Sample output/1
  Generator efficiency compensation/1 -> Limit power to rated/1
  Sample output/1 -> M_g_ref [W]/1
  Zero-Order Hold/1 -> beta_ref [deg]/1
  Limit power to rated/1 -> Region check/3(p_dem), Pitch controller/2(P_dem)
  Region check/1(Torque_ref) -> Saturation/1
  P_dem [W]/1 -> Sample power demand/1
  Torque - speed lookup table/1 -> Region check/1(Torque_dem)  "Desired Torque"
  Saturation/1 -> Rate Limiter/1
  Measurement filter (low pass)/1 -> Sum/2, Region check/2(w_gen), Torque - speed lookup table/1  "Filtered generator speed"
  w_gen_meas [m/s]/1 -> Measurement filter (low pass)/1
  Pitch controller/1(beta_ref [deg]) -> Zero-Order Hold/1, Region check/4(pitch command)
  beta_meas [deg]/1 -> Pitch controller/3(beta_meas [deg])

== system libturbines/Floating IEA15MW/Drive Train ==
  M_rot [Nm] : Inport
  M_gen [Nm] : Inport  Port=2
  Demux : Demux  Outputs=3
  Drive train dynamics : StateSpace  A=wt.dt.ssA  B=wt.dt.ssB  C=wt.dt.ssC  D=wt.dt.ssD  InitialCondition=[wt.rotor.ini;wt.gen.ini;0]
  Mux : Mux  Inputs=2
  w_rot [rad/s] : Outport
  w_gen [rad/s] : Outport  Port=2
  M_shaft [Nm] : Outport  Port=3
  wires:
  Mux/1 -> Drive train dynamics/1
  M_rot [Nm]/1 -> Mux/1
  M_gen [Nm]/1 -> Mux/2
  Drive train dynamics/1 -> Demux/1
  Demux/1 -> w_rot [rad/s]/1
  Demux/2 -> w_gen [rad/s]/1
  Demux/3 -> M_shaft [Nm]/1

== system libturbines/Floating IEA15MW/Generator simple ==
  w_gen [rad/s] : Inport
  M_g_ref [W] : Inport  Port=2
  Constant : Constant  Value=wt.gen.timeconstant
  Divide1 : Product  Inputs=*/
  Generator efficiency : Gain  Gain=wt.gen.effeciency
  Multiply : Product  Inputs=**
  Sum : Sum  Inputs=|+-
  Torque Integrator : Integrator  InitialCondition=wt.gen.torq.ini
  M_gen [Nm] : Outport
  P_out [W] : Outport  Port=2
  wires:
  Constant/1 -> Divide1/2
  Divide1/1 -> Torque Integrator/1
  Generator efficiency/1 -> P_out [W]/1
  Multiply/1 -> Generator efficiency/1
  M_g_ref [W]/1 -> Sum/1
  w_gen [rad/s]/1 -> Multiply/2
  Torque Integrator/1 -> M_gen [Nm]/1, Sum/2, Multiply/1
  Sum/1 -> Divide1/1

== system libturbines/Floating IEA15MW/Hydrodynamics ==
  F_t [N] : Inport
  F_ex : Inport  Port=2
  Gain : Gain  Gain=plat.nF2pT  Multiplication=Matrix(K*u)
  Gain2 : Gain  Gain=plat.pM2nM_surge  Multiplication=Matrix(K*u)
  Gain3 : Gain  Gain=plat.pM2nM_pitch  Multiplication=Matrix(K*u)
  Platform hydrodynamics SS system : StateSpace  A=plat.HydSys.a  B=plat.HydSys.b  C=plat.HydSys.c  D=plat.HydSys.d  InitialCondition=0
  Sum : Sum  Inputs=++|
  Sum2 : Sum  Inputs=+|+
  v_nac_hyd [m/s] : Outport
  wires:
  F_ex/1 -> Sum/2
  Sum/1 -> Platform hydrodynamics SS system/1
  Sum2/1 -> v_nac_hyd [m/s]/1
  Platform hydrodynamics SS system/1 -> Gain3/1, Gain2/1
  Gain2/1 -> Sum2/1
  Gain3/1 -> Sum2/2
  Gain/1 -> Sum/1
  F_t [N]/1 -> Gain/1

== system libturbines/Floating IEA15MW/Pitch Actuator ==
  beta_ref [deg] : Inport
  Pitch system : StateSpace  A=wt.pitch.ssA  B=wt.pitch.ssB  C=wt.pitch.ssC  D=wt.pitch.ssD  InitialCondition=0
  beta [deg] : Outport
  wires:
  beta_ref [deg]/1 -> Pitch system/1
  Pitch system/1 -> beta [deg]/1

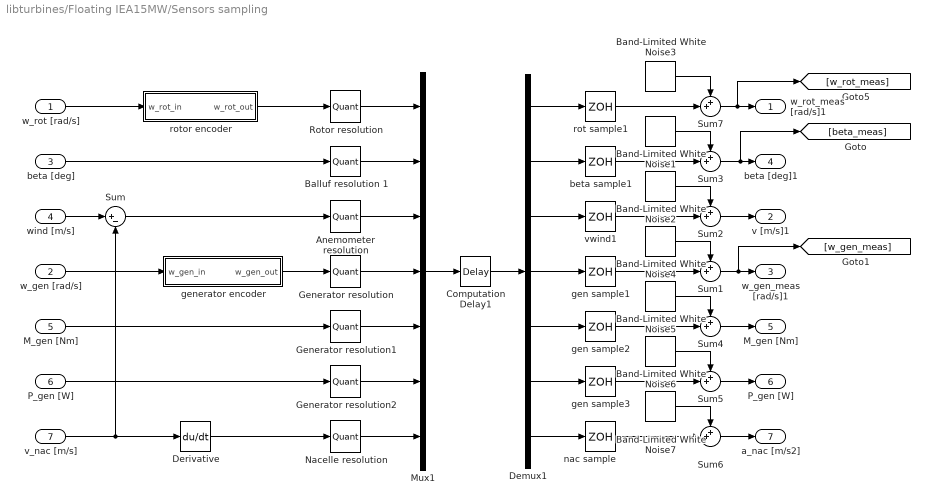
== system libturbines/Floating IEA15MW/Sensors sampling ==
  "w_rot [rad/s] " : Inport
  w_gen [rad/s] : Inport  Port=2
  "beta [deg] " : Inport  Port=3
  wind [m/s] : Inport  Port=4
  "M_gen [Nm] " : Inport  Port=5
  "P_gen [W] " : Inport  Port=6
  "v_nac [m/s] " : Inport  Port=7
  Anemometer resolution : Quantizer  QuantizationInterval=wt.meas.aneres
  Balluf resolution 1 : Quantizer  QuantizationInterval=wt.meas.pitchres
  Band-Limited White Noise1 : simulink/Sources/Band-Limited White Noise  Cov=noiseFlag*wt.meas.pitchnoise  Ts=dt  seed=floor(10000*rand(1))
  Band-Limited White Noise2 : simulink/Sources/Band-Limited White Noise  Cov=noiseFlag*wt.meas.anenoise  Ts=dt  seed=floor(10000*rand(1))
  Band-Limited White Noise3 : simulink/Sources/Band-Limited White Noise  Cov=noiseFlag*wt.meas.rotSpdnoise  Ts=dt  seed=floor(10000*rand(1))
  Band-Limited White Noise4 : simulink/Sources/Band-Limited White Noise  Cov=noiseFlag*wt.meas.genSpdnoise  Ts=dt  seed=floor(10000*rand(1))
  Band-Limited White Noise5 : simulink/Sources/Band-Limited White Noise  Cov=noiseFlag*wt.meas.genTrqnoise  Ts=dt  seed=floor(10000*rand(1))
  Band-Limited White Noise6 : simulink/Sources/Band-Limited White Noise  Cov=noiseFlag*wt.meas.genPwrnoise  Ts=dt  seed=floor(10000*rand(1))
  Band-Limited White Noise7 : simulink/Sources/Band-Limited White Noise  Cov=noiseFlag*wt.meas.nacAccnoise  Ts=dt  seed=floor(10000*rand(1))
  Computation Delay1 : TransportDelay  DelayTime=wt.meas.delay  InitialOutput=[wt.rotor.ini wt.pitch.ini 0 wt.gen.ini 0 0 0]
  Demux1 : Demux  Outputs=7
  Derivative : Derivative
  Generator resolution : Quantizer  QuantizationInterval=wt.meas.genres
  Generator resolution1 : Quantizer  QuantizationInterval=wt.meas.genres
  Generator resolution2 : Quantizer  QuantizationInterval=wt.meas.genres
  Mux1 : Mux  Inputs=7
  Nacelle resolution : Quantizer  QuantizationInterval=wt.meas.nacres
  Rotor resolution : Quantizer  QuantizationInterval=wt.meas.rotres
  Sum : Sum  Inputs=|+-
  Sum{1..7} (7 alike) : Sum  Inputs=++|
  beta sample1 : ZeroOrderHold  SampleTime=wt.meas.Ts
  gen sample1 : ZeroOrderHold  SampleTime=wt.meas.Ts
  gen sample2 : ZeroOrderHold  SampleTime=wt.meas.Ts
  gen sample3 : ZeroOrderHold  SampleTime=wt.meas.Ts
  generator encoder : Subsystem
  nac sample : ZeroOrderHold  SampleTime=wt.meas.Ts
  rot sample1 : ZeroOrderHold  SampleTime=wt.meas.Ts
  rotor encoder : Subsystem
  vwind1 : ZeroOrderHold  SampleTime=wt.meas.Ts
  w_rot_meas [rad/s]1 : Outport  InitialOutput=0
  v [m/s]1 : Outport  Port=2  InitialOutput=0
  w_gen_meas [rad/s]1 : Outport  Port=3  InitialOutput=0
  beta [deg]1 : Outport  Port=4  InitialOutput=0
  M_gen [Nm] : Outport  Port=5  InitialOutput=0
  P_gen [W] : Outport  Port=6  InitialOutput=0
  a_nac [m/s2] : Outport  Port=7  InitialOutput=0
  wires:
  Sum/1 -> Anemometer resolution/1
  wind [m/s]/1 -> Sum/1
  "M_gen [Nm] "/1 -> Generator resolution1/1
  "P_gen [W] "/1 -> Generator resolution2/1
  Derivative/1 -> Nacelle resolution/1
  Nacelle resolution/1 -> Mux1/7
  Generator resolution2/1 -> Mux1/6
  Generator resolution1/1 -> Mux1/5
  Demux1/3 -> vwind1/1
  Demux1/4 -> gen sample1/1
  Demux1/5 -> gen sample2/1
  Demux1/6 -> gen sample3/1
  Demux1/7 -> nac sample/1
  "v_nac [m/s] "/1 -> Derivative/1, Sum/2
  Generator resolution/1 -> Mux1/4
  Anemometer resolution/1 -> Mux1/3
  Balluf resolution 1/1 -> Mux1/2
  Band-Limited White Noise2/1 -> Sum2/1
  gen sample2/1 -> Sum4/2
  Sum1/1 -> w_gen_meas [rad/s]1/1, [w_gen_meas]
  Sum5/1 -> P_gen [W]/1
  gen sample3/1 -> Sum5/2
  Band-Limited White Noise1/1 -> Sum3/1
  nac sample/1 -> Sum6/2
  Sum4/1 -> M_gen [Nm]/1
  Sum6/1 -> a_nac [m/s2]/1
  vwind1/1 -> Sum2/2
  Sum7/1 -> w_rot_meas [rad/s]1/1, [w_rot_meas]
  Band-Limited White Noise4/1 -> Sum1/1
  Band-Limited White Noise5/1 -> Sum4/1
  gen sample1/1 -> Sum1/2
  Band-Limited White Noise3/1 -> Sum7/1
  rot sample1/1 -> Sum7/2
  Mux1/1 -> Computation Delay1/1
  Sum3/1 -> beta [deg]1/1, [beta_meas]
  Sum2/1 -> v [m/s]1/1
  Band-Limited White Noise6/1 -> Sum5/1
  Band-Limited White Noise7/1 -> Sum6/1
  Demux1/2 -> beta sample1/1
  Demux1/1 -> rot sample1/1
  beta sample1/1 -> Sum3/2
  Computation Delay1/1 -> Demux1/1
  "beta [deg] "/1 -> Balluf resolution 1/1
  Rotor resolution/1 -> Mux1/1
  generator encoder/1(w_gen_out) -> Generator resolution/1
  w_gen [rad/s]/1 -> generator encoder/1(w_gen_in)
  "w_rot [rad/s] "/1 -> rotor encoder/1(w_rot_in)
  rotor encoder/1(w_rot_out) -> Rotor resolution/1

== system libturbines/Floating IEA15MW/Tower  ==
  F_t [N] : Inport
  F_t*h : Gain  Gain=wt.tower.height  SaturateOnIntegerOverflow=on  OutDataTypeStr=Inherit: Same as input  ParamDataTypeStr=Inherit: Same as input
  Tower1 : Subsystem  mask(Tower (thrustwise)){mtop=wt.top.mass, mtow=wt.tower.mass, ftowY=wt.tower.eigfreq, dampY=wt.tower.damp}
      mask prompts: mtop "Mass of towertop [kg]"; mtow "Aequivalent tower mass [kg]"; ftowY "Tower eigenfrequency [Hz]"; dampY "Damping coefficient"
      mask help: Thrustwise dynamics of the tower
      mask init:
      | A = [-4*pi*dampY*ftowY,  -4*pi^2*ftowY^2  ; ...
      |                     1                               0       ];
      | B = [1/(mtop+mtow) ; ...
      |           0];
      | C = [1 0 ; ...
      |     0 -4*pi^2*ftowY^2*(mtop+mtow)];
      | D = zeros(2,1);
      mask Help: The thrustwise tower dynamics are modelled as a linear oscillator
  M_tow [Nm] : Outport
  v_nac [m/s] : Outport  Port=2
  wires:
  Tower1/2(F_tow [N]) -> F_t*h/1
  F_t*h/1 -> M_tow [Nm]/1
  F_t [N]/1 -> Tower1/1(FT [Nm])
  Tower1/1(vnac [m/s]) -> v_nac [m/s]/1

== system libturbines/Floating IEA15MW faulty/Aerodynamics ==
  w_rot [rad/s] : Inport
  beta [deg] : Inport  Port=2
  v_rot [m/s] : Inport  Port=3
  Blade 1 : Subsystem
  Blade 2 : Subsystem  AncestorBlock=libturbines/Floating faulty NREL5MW1/Aerodynamics/Blade 1
  Blade 3 : Subsystem  AncestorBlock=libturbines/Floating faulty NREL5MW1/Aerodynamics/Blade 1
  Demux : Demux  Outputs=3
  Sum : Sum  Inputs=+++
  Sum1 : Sum  Inputs=+++
  Sum2 : Sum  Inputs=+++
  M_rot [Nm] : Outport
  F_t [N] : Outport  Port=2
  C_T : Outport  Port=3
  wires:
  Demux/2 -> Blade 2/2(beta [deg])
  Demux/3 -> Blade 3/2(beta [deg])
  Demux/1 -> Blade 1/2(beta [deg])
  beta [deg]/1 -> Demux/1
  Blade 2/2(C_T) -> Sum1/2
  Blade 2/1(F_t [N]) -> Sum/2
  Blade 1/2(C_T) -> Sum1/1
  Blade 1/1(F_t [N]) -> Sum/1
  Blade 1/3(M_rot [Nm]) -> Sum2/1
  Blade 3/2(C_T) -> Sum1/3
  Blade 3/1(F_t [N]) -> Sum/3
  Blade 3/3(M_rot [Nm]) -> Sum2/3
  Blade 2/3(M_rot [Nm]) -> Sum2/2
  Sum1/1 -> C_T/1
  Sum2/1 -> M_rot [Nm]/1
  Sum/1 -> F_t [N]/1
  w_rot [rad/s]/1 -> Blade 1/3(w_rot [rad/s]), Blade 2/3(w_rot [rad/s]), Blade 3/3(w_rot [rad/s])
  v_rot [m/s]/1 -> Blade 1/1(v_rot [m/s]), Blade 2/1(v_rot [m/s]), Blade 3/1(v_rot [m/s])

== system libturbines/Floating IEA15MW faulty/Controller ==
  P_dem [W] : Inport
  w_gen_meas [m/s] : Inport  Port=2
  beta_meas [deg] : Inport  Port=3
  Gain : Gain  Gain=[1 0 0]  Multiplication=Matrix(K*u) (u vector)
  Generator efficiency compensation : Gain  Gain=1/wt.ctrl.gen.effeciency
  Limit power to rated : Saturate  UpperLimit=wt.ctrl.p_rated  LowerLimit=0
  Measurement filter (low pass) : DiscreteStateSpace  A=wt.ctrl.alpha  B=1-wt.ctrl.alpha  C=wt.ctrl.alpha  D=1-wt.ctrl.alpha  InitialCondition=wt.ctrl.gen.ini  SampleTime=wt.ctrl.Ts
  Pitch controller : Subsystem  TreatAsAtomicUnit=on
  Rate Limiter : RateLimiter  RisingSlewLimit=wt.ctrl.torq.ratelim  FallingSlewLimit=-wt.ctrl.torq.ratelim  SampleTimeMode=inherited  InitialCondition=wt.ctrl.torq.ini
  Rated speed : Constant  Value=wt.ctrl.gen.rated
  Region check : Subsystem
  Sample output : ZeroOrderHold  SampleTime=wt.ctrl.Ts
  Sample power demand : ZeroOrderHold  SampleTime=wt.ctrl.Ts
  Saturation : Saturate  UpperLimit=wt.ctrl.torq.lim  LowerLimit=0
  Sum : Sum  Inputs=+-|
  Torque - speed lookup table : Lookup  InputValues=wt.ctrl.torq.wg  Table=wt.ctrl.torq.M  LookUpMeth=Interpolation-Use End Values  SaturateOnIntegerOverflow=off
  Zero-Order Hold : ZeroOrderHold  SampleTime=wt.ctrl.Ts
  beta_ref [deg] : Outport
  T_g_ref [W] : Outport  Port=2
  wires:
  beta_meas [deg]/1 -> Pitch controller/3(beta_meas [deg])
  Gain/1 -> Region check/4(pitch command)
  w_gen_meas [m/s]/1 -> Measurement filter (low pass)/1
  Measurement filter (low pass)/1 -> Torque - speed lookup table/1, Region check/2(w_gen), Sum/2  "Filtered generator speed"
  Saturation/1 -> Rate Limiter/1
  Pitch controller/1(beta_ref [deg]) -> Zero-Order Hold/1, Gain/1
  Torque - speed lookup table/1 -> Region check/1(Torque_dem)  "Desired Torque"
  P_dem [W]/1 -> Sample power demand/1
  Region check/1(Torque_ref) -> Saturation/1
  Limit power to rated/1 -> Pitch controller/2(P_dem), Region check/3(p_dem)
  Zero-Order Hold/1 -> beta_ref [deg]/1
  Sample output/1 -> T_g_ref [W]/1
  Generator efficiency compensation/1 -> Limit power to rated/1
  Rate Limiter/1 -> Sample output/1
  Sample power demand/1 -> Generator efficiency compensation/1
  Rated speed/1 -> Sum/1
  Sum/1 -> Pitch controller/1(w_gen_diff)
  Region check/2(Enable pitch controller) -> Pitch controller/Enable

== system libturbines/Floating IEA15MW faulty/Drive Train ==
  M_rot [Nm] : Inport
  M_gen [Nm] : Inport  Port=2
  Demux : Demux  Outputs=3
  Drive train dynamics : StateSpace  A=wt.dt.ssA  B=wt.dt.ssB  C=wt.dt.ssC  D=wt.dt.ssD  InitialCondition=[wt.rotor.ini;wt.gen.ini;0]
  Mux : Mux  Inputs=2
  w_rot [rad/s] : Outport
  w_gen [rad/s] : Outport  Port=2
  M_shaft [Nm] : Outport  Port=3
  wires:
  Demux/3 -> M_shaft [Nm]/1
  Demux/2 -> w_gen [rad/s]/1
  Demux/1 -> w_rot [rad/s]/1
  Drive train dynamics/1 -> Demux/1
  M_gen [Nm]/1 -> Mux/2
  M_rot [Nm]/1 -> Mux/1
  Mux/1 -> Drive train dynamics/1

== system libturbines/Floating IEA15MW faulty/Generator simple ==
  w_gen [rad/s] : Inport
  T_g_ref [W] : Inport  Port=2
  GenActFault : Inport  Port=3
  Constant : Constant  Value=wt.gen.timeconstant
  Delay : Delay  DelayLength=1  InitialCondition=0
  Delay1 : Delay  DelayLength=1  InitialCondition=0
  Demux : Demux  Outputs=2
  Divide1 : Product  Inputs=*/
  Generator efficiency : Gain  Gain=wt.gen.effeciency
  Generator fault : MATLAB Function  TreatAsAtomicUnit=on
  Generator fault type 3 : MATLAB Function  TreatAsAtomicUnit=on
  Multiply : Product  Inputs=**
  Product : Product
  Sum : Sum  Inputs=|+-
  Torque Integrator : Integrator  InitialCondition=wt.gen.torq.ini
  M_gen [Nm] : Outport
  P_out [W] : Outport  Port=2
  wires:
  Delay1/1 -> Generator fault/4(drift_aux_in)
  Generator fault/2(drift_aux_out) -> Delay1/1
  Delay/1 -> Generator fault/3(torque_prev)
  Sum/1 -> Divide1/1
  Product/1 -> Divide1/2
  Demux/2 -> Product/1
  Constant/1 -> Product/2
  Generator fault/1(torque_real) -> M_gen [Nm]/1, Delay/1, Multiply/1
  Demux/1 -> Generator fault/1(GenActFault)
  Generator fault type 3/1(out) -> Demux/1
  GenActFault/1 -> Generator fault type 3/1(GenActFault)
  w_gen [rad/s]/1 -> Multiply/2
  Torque Integrator/1 -> Sum/2, Generator fault/2(torque)
  T_g_ref [W]/1 -> Sum/1
  Multiply/1 -> Generator efficiency/1
  Generator efficiency/1 -> P_out [W]/1
  Divide1/1 -> Torque Integrator/1

== system libturbines/Floating IEA15MW faulty/Hydrodynamics ==
  F_t [N] : Inport
  F_ex : Inport  Port=2
  Gain : Gain  Gain=plat.nF2pT  Multiplication=Matrix(K*u)
  Gain2 : Gain  Gain=plat.pM2nM_surge  Multiplication=Matrix(K*u)
  Gain3 : Gain  Gain=plat.pM2nM_pitch  Multiplication=Matrix(K*u)
  Platform hydrodynamics SS system : StateSpace  A=plat.HydSys.a  B=plat.HydSys.b  C=plat.HydSys.c  D=plat.HydSys.d  InitialCondition=0
  Sum : Sum  Inputs=++|
  Sum2 : Sum  Inputs=+|+
  v_nac_hyd [m/s] : Outport
  wires:
  F_t [N]/1 -> Gain/1
  Gain/1 -> Sum/1
  Gain3/1 -> Sum2/2
  Gain2/1 -> Sum2/1
  Platform hydrodynamics SS system/1 -> Gain2/1, Gain3/1
  Sum2/1 -> v_nac_hyd [m/s]/1
  Sum/1 -> Platform hydrodynamics SS system/1
  F_ex/1 -> Sum/2

== system libturbines/Floating IEA15MW faulty/Pitch Actuator ==
  beta_ref [deg] : Inport
  PitchActFault : Inport  Port=2
  Delay1 : Delay  DelayLength=1  InitialCondition=0
  Delay2 : Delay  DelayLength=1  InitialCondition=0
  Pitch actuator fault : MATLAB Function  TreatAsAtomicUnit=on
  Pitch subsystems : Subsystem
  beta [deg] : Outport
  wires:
  Delay1/1 -> Pitch actuator fault/2(beta_prev)
  Delay2/1 -> Pitch actuator fault/4(drift_aux_in)
  Pitch actuator fault/2(drift_aux_out) -> Delay2/1
  Pitch subsystems/1(beta [deg]) -> Pitch actuator fault/1(beta)
  Pitch actuator fault/1(beta_real) -> beta [deg]/1, Delay1/1
  beta_ref [deg]/1 -> Pitch subsystems/1(beta_ref [deg])
  PitchActFault/1 -> Pitch actuator fault/3(PitchActFault), Pitch subsystems/2(Fault type 5)
